simulink model "simu_starting_program23"  (R2023b)
settings: Solver=FixedStepAuto  StartTime=0.0  StopTime=6  RelTol=1e-3
StartFcn:
  | MaxMissedTicks = 99^100;
  | SampleTime = 0.01;
undefined symbols (not defined in the file or in its folder): National_Instruments, PCI
libraries: sldrtlib x24, simulink x2, simulink_extras x2
settings Model: Creator=labadmin  LastModifiedBy=aie4-26
settings HardwareCC: ProdBitPerLong=64  ProdHWDeviceType=Intel->x86-64 (Linux 64)
settings RTWCC: Description=Simulink Desktop Real-Time  SystemTargetFile=sldrt.tlc  TemplateMakefile=sldrt.tmf  RTWCompilerOptimization=on
settings CodeAppCC: MaxIdLength=95
settings SimulinkDesktopRealTimeCC: TargetLibSuffix=_sldrt.a  TargetPreCompLibLocation=C:\Program Files\MATLAB\R2025b\toolbox\sldrt\lib\win64  ParMdlRefBuildCompliant=on
settings ConfigComp: CovBoundaryAbsTol=1.0e-5

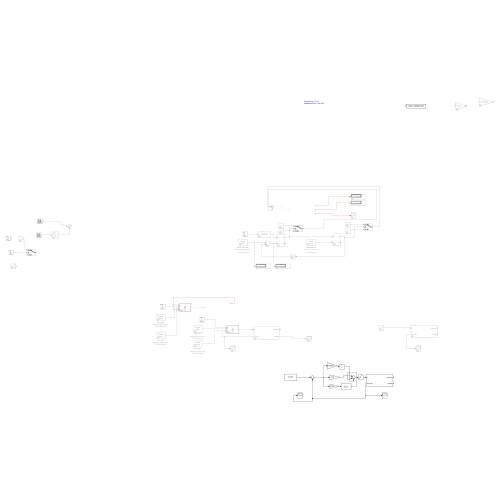
[thumbnail: Simulink's stored preview of the top-level diagram]
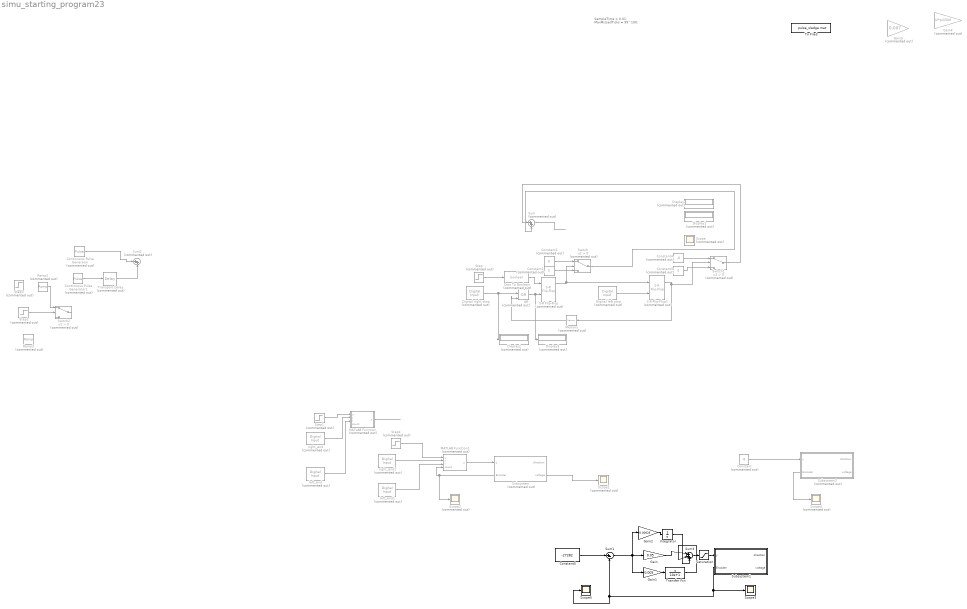
== system simu_starting_program23 ==
  note: SampleTime = 0.01;
      | MaxMissedTicks = 99^100;
  Cast To Boolean : DataTypeConversion  Commented=on  OutDataTypeStr=boolean  SaturateOnIntegerOverflow=off  RndMeth=Floor
  Constant : Constant  Commented=on  Value=-8
  Constant1 : Constant  Commented=on  Value=8
  Constant2 : Constant  Commented=on  Value=0
  Constant3 : Constant  Commented=on  Value=0
  Constant4 : Constant  Commented=on  Value=-8
  Constant5 : Constant  Value=-27282
  Continuous Pulse Generator : DiscretePulseGenerator  Commented=on  PulseType=Time based  Amplitude=1.8  Period=20  PulseWidth=5
  Continuous Pulse Generator1 : DiscretePulseGenerator  Commented=on  PulseType=Time based  Amplitude=-1.8  Period=20  PulseWidth=5
  Digital left stop : sldrtlib/Digital Input  Commented=on  SampleTime=0.1  MaxMissedTicks=10  ShowMissedTicks=off  YieldWhenWaiting=off  DrvName=National_Instruments/PCI-6229  DrvAddress=4294967295  DrvOptions=[1 1 8192 2 3]  Channels=2  BitMode=1  DataType=9
      settings: AttributesFormatString=National Instruments\nPCI-6229 [auto]
  Digital right stop : sldrtlib/Digital Input  Commented=on  SampleTime=0.1  MaxMissedTicks=10  ShowMissedTicks=off  YieldWhenWaiting=off  DrvName=National_Instruments/PCI-6229  DrvAddress=4294967295  DrvOptions=[1 1 8192 2 3]  Channels=3  BitMode=1  DataType=9
      settings: AttributesFormatString=National Instruments\nPCI-6229 [auto]
  Display{,1..3} (4 alike) : Display  Commented=on
  Gain : Gain  Gain=0.05
  Gain1 : Gain  Gain=0.005
  Gain2 : Gain  Gain=0.00026
  Gain4 : Gain  Commented=on  Gain=(2*pi)/500
  Gain5 : Gain  Commented=on  Gain=0.007
  Integrator : Integrator
  MATLAB Function : MATLAB Function  Commented=on  TreatAsAtomicUnit=on
  MATLAB Function1 : MATLAB Function  Commented=on  TreatAsAtomicUnit=on
  Memory : Memory  Commented=on
  OR : Logic  Commented=on  Operator=OR  IconShape=distinctive  AllPortsSameDT=off  OutDataTypeStr=boolean
  Ramp2 : simulink/Sources/Ramp  Commented=on  slope=-2  start=0  InitialOutput=0
  Ramp3 : simulink/Sources/Ramp  Commented=on  slope=1.5  start=7  InitialOutput=0
  S-R Flip-Flop : simulink_extras/Flip Flops/S-R Flip-Flop  Commented=on  initial_condition=0
  S-R Flip-Flop1 : simulink_extras/Flip Flops/S-R Flip-Flop  Commented=on  initial_condition=0
  Saturation : Saturate  UpperLimit=10  LowerLimit=-10
  Scope{,1..2,4} (4 alike) : Scope  Commented=on
  Scope3 : Scope
  Scope5 : Scope
  Step : Step  Commented=on  Before=1  After=0  SampleTime=0
  Step1 : Step  Commented=on  Before=1  After=0  SampleTime=0
  Step2 : Step  Commented=on  Time=6  Before=1  After=0  SampleTime=0
  Step3 : Step  Commented=on  Time=6  Before=1  After=0  SampleTime=0
  Step4 : Step  Commented=on  Before=1  After=0  SampleTime=0
  Subsystem : Subsystem  Commented=on
      settings: PortSchema="{\"entries\":[{\"content\":{\"sides\":[{\"content\":{\"connectorIds\":[\"In1\",\"Out3\"]},\"type\":\"ConnectorPlacement.EquallySpacedRectSide\",\"uuid\":\"4cea31ae-feeb-4317-b838-0a7fffa1c8c1\"},{\"content\":{\"connectorIds\":[\"Out1\",\"Out2\"],\"side\":\"RIGHT\"},\"type\":\"ConnectorPlacement.EquallySpacedRectSide\",\"uuid\":\"cbbf0856-f885-4a01-8596-30b50a35b1ee\"},{\"content\":{\"side\":\"TOP\"},\"type\":\"ConnectorPlacement.EquallySpacedRectSide\",\"uuid\":\"67ac1927-d07b-45dd-8475-804e77d14220\"}]},\"type\":\"ConnectorPlacement.EquallySpacedConnector\",\"uuid\":\"0da884d4-170d-4ce1-a87a-0ec272783a4a\"}],\"packageUris\":[\"http://schema.mathworks.com/mf0/Connector/R2020b\"],\"version\":\"1.0\"}"
  Subsystem1 : Subsystem
      settings: PortSchema="{\"entries\":[{\"content\":{\"sides\":[{\"content\":{\"connectorIds\":[\"In1\",\"Out3\"]},\"type\":\"ConnectorPlacement.EquallySpacedRectSide\",\"uuid\":\"4cea31ae-feeb-4317-b838-0a7fffa1c8c1\"},{\"content\":{\"connectorIds\":[\"Out1\",\"Out2\"],\"side\":\"RIGHT\"},\"type\":\"ConnectorPlacement.EquallySpacedRectSide\",\"uuid\":\"cbbf0856-f885-4a01-8596-30b50a35b1ee\"},{\"content\":{\"side\":\"TOP\"},\"type\":\"ConnectorPlacement.EquallySpacedRectSide\",\"uuid\":\"67ac1927-d07b-45dd-8475-804e77d14220\"}]},\"type\":\"ConnectorPlacement.EquallySpacedConnector\",\"uuid\":\"0da884d4-170d-4ce1-a87a-0ec272783a4a\"}],\"packageUris\":[\"http://schema.mathworks.com/mf0/Connector/R2020b\"],\"version\":\"1.0\"}"
  Subsystem2 : Subsystem  Commented=on
      settings: PortSchema="{\"entries\":[{\"content\":{\"sides\":[{\"content\":{\"connectorIds\":[\"In1\",\"Out3\"]},\"type\":\"ConnectorPlacement.EquallySpacedRectSide\",\"uuid\":\"4cea31ae-feeb-4317-b838-0a7fffa1c8c1\"},{\"content\":{\"connectorIds\":[\"Out1\",\"Out2\"],\"side\":\"RIGHT\"},\"type\":\"ConnectorPlacement.EquallySpacedRectSide\",\"uuid\":\"cbbf0856-f885-4a01-8596-30b50a35b1ee\"},{\"content\":{\"side\":\"TOP\"},\"type\":\"ConnectorPlacement.EquallySpacedRectSide\",\"uuid\":\"67ac1927-d07b-45dd-8475-804e77d14220\"}]},\"type\":\"ConnectorPlacement.EquallySpacedConnector\",\"uuid\":\"0da884d4-170d-4ce1-a87a-0ec272783a4a\"}],\"packageUris\":[\"http://schema.mathworks.com/mf0/Connector/R2020b\"],\"version\":\"1.0\"}"
  Sum : Sum  Commented=on  Inputs=|++
  Sum1 : Sum  Inputs=|+-
  Sum2 : Sum  Commented=on  Inputs=|++
  Sum3 : Sum  Inputs=|+++
  Switch : Switch  Commented=on  Criteria=u2 > Threshold  SaturateOnIntegerOverflow=off  InputSameDT=off
  Switch1 : Switch  Commented=on  Criteria=u2 > Threshold  SaturateOnIntegerOverflow=off  InputSameDT=off
  Switch2 : Switch  Commented=on  Criteria=u2 > Threshold  SaturateOnIntegerOverflow=off  InputSameDT=off
  To File3 : ToFile  Filename=pulse_sledge.mat  SaveFormat=Timeseries
  Transfer Fcn : TransferFcn  Numerator=[1 0 ]  Denominator=[10 1]
  Transport Delay : TransportDelay  Commented=on  DelayTime=10
  left_end : sldrtlib/Digital Input  Commented=on  SampleTime=0.1  MaxMissedTicks=10  ShowMissedTicks=off  YieldWhenWaiting=off  DrvName=National_Instruments/PCI-6229  DrvAddress=4294967295  DrvOptions=[1 1 8192 2 3]  Channels=2  BitMode=1  DataType=1
      settings: AttributesFormatString=National Instruments\nPCI-6229 [auto]
  left_end1 : sldrtlib/Digital Input  Commented=on  SampleTime=0.1  MaxMissedTicks=10  ShowMissedTicks=off  YieldWhenWaiting=off  DrvName=National_Instruments/PCI-6229  DrvAddress=4294967295  DrvOptions=[1 1 8192 2 3]  Channels=2  BitMode=1  DataType=9
      settings: AttributesFormatString=National Instruments\nPCI-6229 [auto]
  right_end : sldrtlib/Digital Input  Commented=on  SampleTime=0.1  MaxMissedTicks=10  ShowMissedTicks=off  YieldWhenWaiting=off  DrvName=National_Instruments/PCI-6229  DrvAddress=4294967295  DrvOptions=[1 1 8192 2 3]  Channels=3  BitMode=1  DataType=9
      settings: AttributesFormatString=National Instruments\nPCI-6229 [auto]
  right_end1 : sldrtlib/Digital Input  Commented=on  SampleTime=0.1  MaxMissedTicks=10  ShowMissedTicks=off  YieldWhenWaiting=off  DrvName=National_Instruments/PCI-6229  DrvAddress=4294967295  DrvOptions=[1 1 8192 2 3]  Channels=3  BitMode=1  DataType=9
      settings: AttributesFormatString=National Instruments\nPCI-6229 [auto]
  wires:
  Continuous Pulse Generator1/1 -> Transport Delay/1
  Continuous Pulse Generator/1 -> Sum2/1
  Transport Delay/1 -> Sum2/2
  Ramp2/1 -> Switch2/1
  Step2/1 -> Switch2/2
  ? -> Display/1
  ? -> Display1/1
  ? -> Scope/1
  Step/1 -> Cast To Boolean/1
  Digital right stop/1 -> Display2/1, OR/1
  OR/1 -> Display3/1, S-R Flip-Flop/2
  S-R Flip-Flop1/1 -> Switch1/2, Memory/1
  S-R Flip-Flop/1 -> S-R Flip-Flop1/1, Switch/2
  Switch/1 -> Sum/2
  Constant2/1 -> Switch/3
  Constant1/1 -> Switch/1
  Constant3/1 -> Switch1/3
  Constant4/1 -> Switch1/1
  Switch1/1 -> Sum/1
  Sum/1 -> ?
  Digital left stop/1 -> S-R Flip-Flop1/2
  Cast To Boolean/1 -> S-R Flip-Flop/1
  Memory/1 -> OR/2
  MATLAB Function/1(y) -> ?
  Step1/1 -> MATLAB Function/1(u)
  right_end/1 -> MATLAB Function/2(r)
  left_end/1 -> MATLAB Function/3(l)
  ? -> MATLAB Function/4(count)
  MATLAB Function1/1(y) -> Subsystem/1(y)
  right_end1/1 -> MATLAB Function1/2(r)
  Step4/1 -> MATLAB Function1/1(u)
  left_end1/1 -> MATLAB Function1/3(l)
  Subsystem/2(voltage) -> Scope1/1
  Subsystem/3(Encoder) -> Scope2/1, MATLAB Function1/4(count)
  Constant5/1 -> Sum1/1
  Gain/1 -> Sum3/1
  Gain1/1 -> Transfer Fcn/1
  Sum3/1 -> Saturation/1
  Constant/1 -> Subsystem2/1(y)
  Subsystem2/3(Encoder) -> Scope4/1
  Sum1/1 -> Gain2/1, Gain1/1, Gain/1
  Subsystem1/3(Encoder) -> Sum1/2, Scope5/1, Scope3/1
  Saturation/1 -> Subsystem1/1(y)
  Transfer Fcn/1 -> Sum3/2
  Gain2/1 -> Integrator/1
  Integrator/1 -> Sum3/3

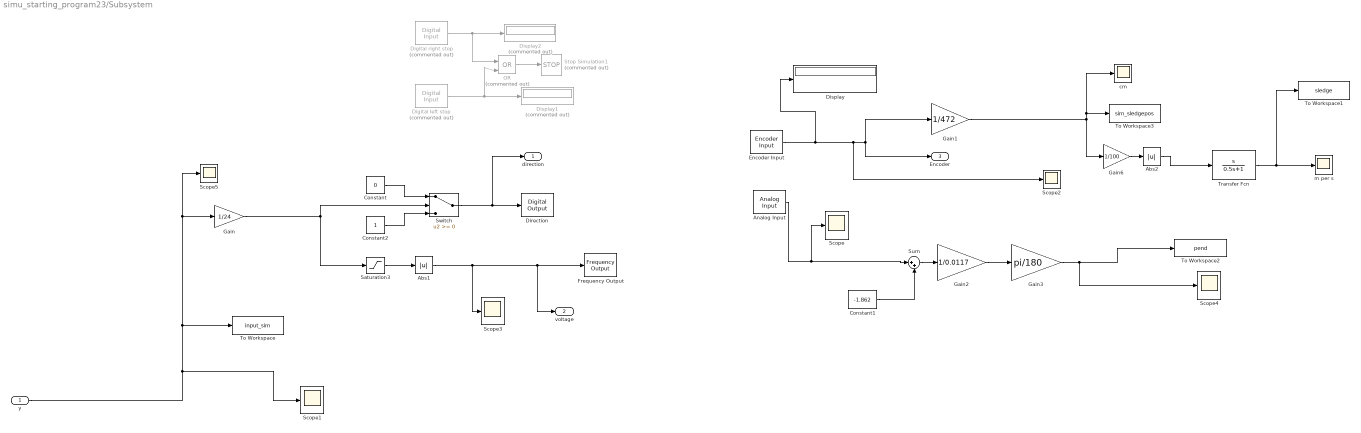
== system simu_starting_program23/Subsystem ==
  y : Inport
  Abs1 : Abs  SaturateOnIntegerOverflow=off
  Abs2 : Abs  SaturateOnIntegerOverflow=off
  Analog Input : sldrtlib/Analog Input  SampleTime=SampleTime  MaxMissedTicks=MaxMissedTicks  ShowMissedTicks=off  YieldWhenWaiting=off  DrvName=National_Instruments/PCI-6229  DrvAddress=4294967295  DrvOptions=[1 1 8192 2 3]  Channels=1  RangeMode=1  VoltRange=1  DataType=1
      settings: AttributesFormatString=National Instruments\nPCI-6229 [auto]
  Constant : Constant  Value=0  SampleTime=SampleTime
  Constant1 : Constant  Value=-1.862
  Constant2 : Constant  SampleTime=SampleTime
  Digital left stop : sldrtlib/Digital Input  Commented=on  SampleTime=0.1  MaxMissedTicks=10  ShowMissedTicks=off  YieldWhenWaiting=off  DrvName=National_Instruments/PCI-6229  DrvAddress=4294967295  DrvOptions=[1 1 8192 2 3]  Channels=2  BitMode=1  DataType=1
      settings: AttributesFormatString=National Instruments\nPCI-6229 [auto]
  Digital right stop : sldrtlib/Digital Input  Commented=on  SampleTime=0.1  MaxMissedTicks=10  ShowMissedTicks=off  YieldWhenWaiting=off  DrvName=National_Instruments/PCI-6229  DrvAddress=4294967295  DrvOptions=[1 1 8192 2 3]  Channels=3  BitMode=1  DataType=9
      settings: AttributesFormatString=National Instruments\nPCI-6229 [auto]
  Direction : sldrtlib/Digital Output  SampleTime=SampleTime  MaxMissedTicks=MaxMissedTicks  ShowMissedTicks=off  YieldWhenWaiting=off  DrvName=National_Instruments/PCI-6229  DrvAddress=4294967295  DrvOptions=[1 1 8192 2 3]  Channels=1  BitMode=1  InitialValue=0  FinalValue=0
      settings: AttributesFormatString=National Instruments\nPCI-6229 [auto]
  Display : Display
  Display1 : Display  Commented=on
  Display2 : Display  Commented=on
  Encoder Input : sldrtlib/Encoder Input  SampleTime=SampleTime  MaxMissedTicks=MaxMissedTicks  ShowMissedTicks=off  YieldWhenWaiting=off  DrvName=National_Instruments/PCI-6229  DrvAddress=4294967295  DrvOptions=[1 1 8192 2 3]  Channels=1  QuadMode=3  IndexPulse=2  InputFilter=Inf  DataType=1
      settings: AttributesFormatString=National Instruments\nPCI-6229 [auto]
  Frequency Output : sldrtlib/Frequency Output  SampleTime=SampleTime  MaxMissedTicks=MaxMissedTicks  ShowMissedTicks=off  YieldWhenWaiting=off  DrvName=National_Instruments/PCI-6229  DrvAddress=4294967295  DrvOptions=[1 1 8192 2 3]  Channels=2  FrequencySource=1  Frequency=10000  FrequencyFinalValue=[]  DutySource=2  Duty=0  DutyFinalValue=0
      settings: AttributesFormatString=National Instruments\nPCI-6229 [auto]
  Gain : Gain  Gain=1/24
  Gain1 : Gain  Gain=1/472
  Gain2 : Gain  Gain=1/0.0117
  Gain3 : Gain  Gain=pi/180
  Gain6 : Gain  Gain=1/100
  OR : Logic  Commented=on  Operator=OR  IconShape=distinctive  AllPortsSameDT=off  OutDataTypeStr=boolean
  Saturation3 : Saturate
  Scope{,1..5} (6 alike) : Scope
  Stop Simulation1 : Stop  Commented=on
  Sum : Sum  Inputs=|++
  Switch : Switch  SaturateOnIntegerOverflow=off  InputSameDT=off
  To Workspace : ToWorkspace  VariableName=input_sim  SaveFormat=Timeseries  SampleTime=-1
  To Workspace1 : ToWorkspace  VariableName=sledge  SaveFormat=Timeseries  SampleTime=-1
  To Workspace2 : ToWorkspace  VariableName=pend  SaveFormat=Timeseries  SampleTime=-1
  To Workspace3 : ToWorkspace  VariableName=sim_sledgepos  SaveFormat=Timeseries  SampleTime=-1
  Transfer Fcn : TransferFcn  Numerator=[1 0]  Denominator=[0.5 1]
  cm : Scope
  m per s : Scope
  direction : Outport
  voltage : Outport  Port=2
  Encoder : Outport  Port=3
  wires:
  Gain1/1 -> Gain6/1, To Workspace3/1, cm/1
  Abs2/1 -> Transfer Fcn/1
  Switch/1 -> direction/1, Direction/1
  Gain2/1 -> Gain3/1
  Digital left stop/1 -> OR/2, Display1/1
  Constant/1 -> Switch/1
  Transfer Fcn/1 -> To Workspace1/1, m per s/1
  y/1 -> To Workspace/1, Scope5/1, Gain/1, Scope1/1
  Gain3/1 -> Scope4/1, To Workspace2/1
  OR/1 -> Stop Simulation1/1
  Digital right stop/1 -> OR/1, Display2/1
  Analog Input/1 -> Sum/1, Scope/1
  Saturation3/1 -> Abs1/1
  Gain/1 -> Saturation3/1, Switch/2
  Gain6/1 -> Abs2/1
  Constant2/1 -> Switch/3
  Sum/1 -> Gain2/1
  Abs1/1 -> Scope3/1, voltage/1, Frequency Output/1
  Constant1/1 -> Sum/2
  Encoder Input/1 -> Display/1, Scope2/1, Encoder/1, Gain1/1

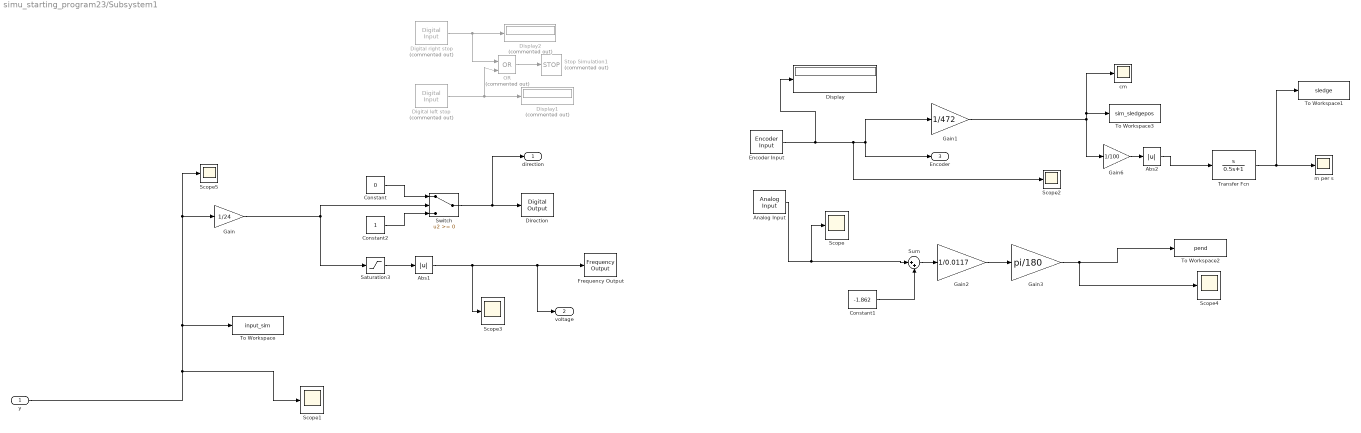
== system simu_starting_program23/Subsystem1 ==
  y : Inport
  Abs1 : Abs  SaturateOnIntegerOverflow=off
  Abs2 : Abs  SaturateOnIntegerOverflow=off
  Analog Input : sldrtlib/Analog Input  SampleTime=SampleTime  MaxMissedTicks=MaxMissedTicks  ShowMissedTicks=off  YieldWhenWaiting=off  DrvName=National_Instruments/PCI-6229  DrvAddress=4294967295  DrvOptions=[1 1 8192 2 3]  Channels=1  RangeMode=1  VoltRange=1  DataType=1
      settings: AttributesFormatString=National Instruments\nPCI-6229 [auto]
  Constant : Constant  Value=0  SampleTime=SampleTime
  Constant1 : Constant  Value=-1.862
  Constant2 : Constant  SampleTime=SampleTime
  Digital left stop : sldrtlib/Digital Input  Commented=on  SampleTime=0.1  MaxMissedTicks=10  ShowMissedTicks=off  YieldWhenWaiting=off  DrvName=National_Instruments/PCI-6229  DrvAddress=4294967295  DrvOptions=[1 1 8192 2 3]  Channels=2  BitMode=1  DataType=1
      settings: AttributesFormatString=National Instruments\nPCI-6229 [auto]
  Digital right stop : sldrtlib/Digital Input  Commented=on  SampleTime=0.1  MaxMissedTicks=10  ShowMissedTicks=off  YieldWhenWaiting=off  DrvName=National_Instruments/PCI-6229  DrvAddress=4294967295  DrvOptions=[1 1 8192 2 3]  Channels=3  BitMode=1  DataType=9
      settings: AttributesFormatString=National Instruments\nPCI-6229 [auto]
  Direction : sldrtlib/Digital Output  SampleTime=SampleTime  MaxMissedTicks=MaxMissedTicks  ShowMissedTicks=off  YieldWhenWaiting=off  DrvName=National_Instruments/PCI-6229  DrvAddress=4294967295  DrvOptions=[1 1 8192 2 3]  Channels=1  BitMode=1  InitialValue=0  FinalValue=0
      settings: AttributesFormatString=National Instruments\nPCI-6229 [auto]
  Display : Display
  Display1 : Display  Commented=on
  Display2 : Display  Commented=on
  Encoder Input : sldrtlib/Encoder Input  SampleTime=SampleTime  MaxMissedTicks=MaxMissedTicks  ShowMissedTicks=off  YieldWhenWaiting=off  DrvName=National_Instruments/PCI-6229  DrvAddress=4294967295  DrvOptions=[1 1 8192 2 3]  Channels=1  QuadMode=3  IndexPulse=2  InputFilter=Inf  DataType=1
      settings: AttributesFormatString=National Instruments\nPCI-6229 [auto]
  Frequency Output : sldrtlib/Frequency Output  SampleTime=SampleTime  MaxMissedTicks=MaxMissedTicks  ShowMissedTicks=off  YieldWhenWaiting=off  DrvName=National_Instruments/PCI-6229  DrvAddress=4294967295  DrvOptions=[1 1 8192 2 3]  Channels=2  FrequencySource=1  Frequency=10000  FrequencyFinalValue=[]  DutySource=2  Duty=0  DutyFinalValue=0
      settings: AttributesFormatString=National Instruments\nPCI-6229 [auto]
  Gain : Gain  Gain=1/24
  Gain1 : Gain  Gain=1/472
  Gain2 : Gain  Gain=1/0.0117
  Gain3 : Gain  Gain=pi/180
  Gain6 : Gain  Gain=1/100
  OR : Logic  Commented=on  Operator=OR  IconShape=distinctive  AllPortsSameDT=off  OutDataTypeStr=boolean
  Saturation3 : Saturate
  Scope{,1..5} (6 alike) : Scope
  Stop Simulation1 : Stop  Commented=on
  Sum : Sum  Inputs=|++
  Switch : Switch  SaturateOnIntegerOverflow=off  InputSameDT=off
  To Workspace : ToWorkspace  VariableName=input_sim  SaveFormat=Timeseries  SampleTime=-1
  To Workspace1 : ToWorkspace  VariableName=sledge  SaveFormat=Timeseries  SampleTime=-1
  To Workspace2 : ToWorkspace  VariableName=pend  SaveFormat=Timeseries  SampleTime=-1
  To Workspace3 : ToWorkspace  VariableName=sim_sledgepos  SaveFormat=Timeseries  SampleTime=-1
  Transfer Fcn : TransferFcn  Numerator=[1 0]  Denominator=[0.5 1]
  cm : Scope
  m per s : Scope
  direction : Outport
  voltage : Outport  Port=2
  Encoder : Outport  Port=3
  wires:
  Encoder Input/1 -> Gain1/1, Encoder/1, Scope2/1, Display/1
  Constant1/1 -> Sum/2
  Abs1/1 -> Frequency Output/1, voltage/1, Scope3/1
  Sum/1 -> Gain2/1
  Constant2/1 -> Switch/3
  Gain6/1 -> Abs2/1
  Gain/1 -> Switch/2, Saturation3/1
  Saturation3/1 -> Abs1/1
  Analog Input/1 -> Scope/1, Sum/1
  Digital right stop/1 -> Display2/1, OR/1
  OR/1 -> Stop Simulation1/1
  Gain3/1 -> To Workspace2/1, Scope4/1
  y/1 -> Scope1/1, Gain/1, Scope5/1, To Workspace/1
  Transfer Fcn/1 -> m per s/1, To Workspace1/1
  Constant/1 -> Switch/1
  Digital left stop/1 -> Display1/1, OR/2
  Gain2/1 -> Gain3/1
  Switch/1 -> Direction/1, direction/1
  Abs2/1 -> Transfer Fcn/1
  Gain1/1 -> cm/1, To Workspace3/1, Gain6/1

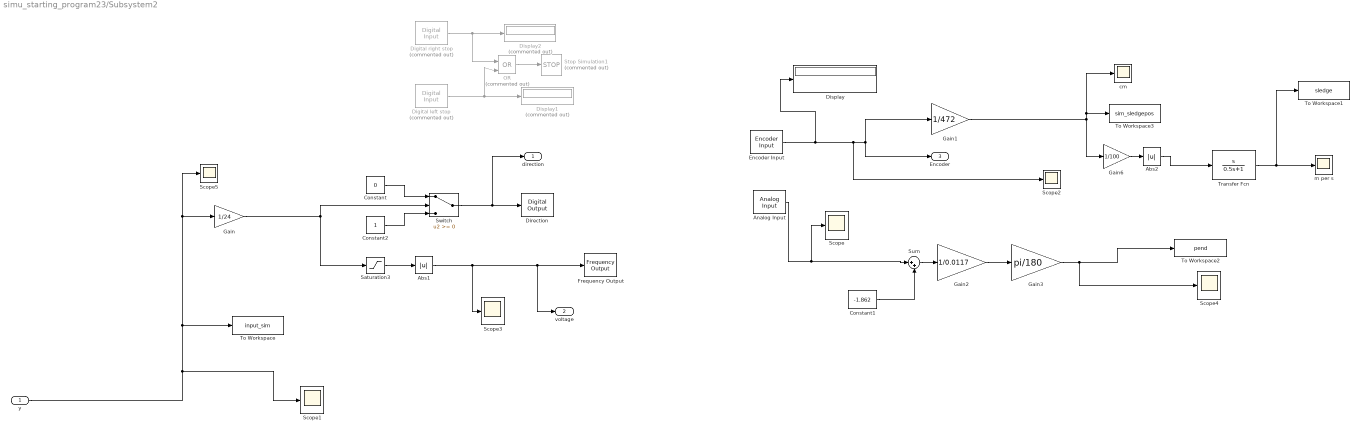
== system simu_starting_program23/Subsystem2 ==
  y : Inport
  Abs1 : Abs  SaturateOnIntegerOverflow=off
  Abs2 : Abs  SaturateOnIntegerOverflow=off
  Analog Input : sldrtlib/Analog Input  SampleTime=SampleTime  MaxMissedTicks=MaxMissedTicks  ShowMissedTicks=off  YieldWhenWaiting=off  DrvName=National_Instruments/PCI-6229  DrvAddress=4294967295  DrvOptions=[1 1 8192 2 3]  Channels=1  RangeMode=1  VoltRange=1  DataType=1
      settings: AttributesFormatString=National Instruments\nPCI-6229 [auto]
  Constant : Constant  Value=0  SampleTime=SampleTime
  Constant1 : Constant  Value=-1.862
  Constant2 : Constant  SampleTime=SampleTime
  Digital left stop : sldrtlib/Digital Input  Commented=on  SampleTime=0.1  MaxMissedTicks=10  ShowMissedTicks=off  YieldWhenWaiting=off  DrvName=National_Instruments/PCI-6229  DrvAddress=4294967295  DrvOptions=[1 1 8192 2 3]  Channels=2  BitMode=1  DataType=1
      settings: AttributesFormatString=National Instruments\nPCI-6229 [auto]
  Digital right stop : sldrtlib/Digital Input  Commented=on  SampleTime=0.1  MaxMissedTicks=10  ShowMissedTicks=off  YieldWhenWaiting=off  DrvName=National_Instruments/PCI-6229  DrvAddress=4294967295  DrvOptions=[1 1 8192 2 3]  Channels=3  BitMode=1  DataType=9
      settings: AttributesFormatString=National Instruments\nPCI-6229 [auto]
  Direction : sldrtlib/Digital Output  SampleTime=SampleTime  MaxMissedTicks=MaxMissedTicks  ShowMissedTicks=off  YieldWhenWaiting=off  DrvName=National_Instruments/PCI-6229  DrvAddress=4294967295  DrvOptions=[1 1 8192 2 3]  Channels=1  BitMode=1  InitialValue=0  FinalValue=0
      settings: AttributesFormatString=National Instruments\nPCI-6229 [auto]
  Display : Display
  Display1 : Display  Commented=on
  Display2 : Display  Commented=on
  Encoder Input : sldrtlib/Encoder Input  SampleTime=SampleTime  MaxMissedTicks=MaxMissedTicks  ShowMissedTicks=off  YieldWhenWaiting=off  DrvName=National_Instruments/PCI-6229  DrvAddress=4294967295  DrvOptions=[1 1 8192 2 3]  Channels=1  QuadMode=3  IndexPulse=2  InputFilter=Inf  DataType=1
      settings: AttributesFormatString=National Instruments\nPCI-6229 [auto]
  Frequency Output : sldrtlib/Frequency Output  SampleTime=SampleTime  MaxMissedTicks=MaxMissedTicks  ShowMissedTicks=off  YieldWhenWaiting=off  DrvName=National_Instruments/PCI-6229  DrvAddress=4294967295  DrvOptions=[1 1 8192 2 3]  Channels=2  FrequencySource=1  Frequency=10000  FrequencyFinalValue=[]  DutySource=2  Duty=0  DutyFinalValue=0
      settings: AttributesFormatString=National Instruments\nPCI-6229 [auto]
  Gain : Gain  Gain=1/24
  Gain1 : Gain  Gain=1/472
  Gain2 : Gain  Gain=1/0.0117
  Gain3 : Gain  Gain=pi/180
  Gain6 : Gain  Gain=1/100
  OR : Logic  Commented=on  Operator=OR  IconShape=distinctive  AllPortsSameDT=off  OutDataTypeStr=boolean
  Saturation3 : Saturate
  Scope{,1..5} (6 alike) : Scope
  Stop Simulation1 : Stop  Commented=on
  Sum : Sum  Inputs=|++
  Switch : Switch  SaturateOnIntegerOverflow=off  InputSameDT=off
  To Workspace : ToWorkspace  VariableName=input_sim  SaveFormat=Timeseries  SampleTime=-1
  To Workspace1 : ToWorkspace  VariableName=sledge  SaveFormat=Timeseries  SampleTime=-1
  To Workspace2 : ToWorkspace  VariableName=pend  SaveFormat=Timeseries  SampleTime=-1
  To Workspace3 : ToWorkspace  VariableName=sim_sledgepos  SaveFormat=Timeseries  SampleTime=-1
  Transfer Fcn : TransferFcn  Numerator=[1 0]  Denominator=[0.5 1]
  cm : Scope
  m per s : Scope
  direction : Outport
  voltage : Outport  Port=2
  Encoder : Outport  Port=3
  wires:
  Gain1/1 -> Gain6/1, To Workspace3/1, cm/1
  Abs2/1 -> Transfer Fcn/1
  Switch/1 -> direction/1, Direction/1
  Gain2/1 -> Gain3/1
  Digital left stop/1 -> OR/2, Display1/1
  Constant/1 -> Switch/1
  Transfer Fcn/1 -> To Workspace1/1, m per s/1
  y/1 -> To Workspace/1, Scope5/1, Gain/1, Scope1/1
  Gain3/1 -> Scope4/1, To Workspace2/1
  OR/1 -> Stop Simulation1/1
  Digital right stop/1 -> OR/1, Display2/1
  Analog Input/1 -> Sum/1, Scope/1
  Saturation3/1 -> Abs1/1
  Gain/1 -> Saturation3/1, Switch/2
  Gain6/1 -> Abs2/1
  Constant2/1 -> Switch/3
  Sum/1 -> Gain2/1
  Abs1/1 -> Scope3/1, voltage/1, Frequency Output/1
  Constant1/1 -> Sum/2
  Encoder Input/1 -> Display/1, Scope2/1, Encoder/1, Gain1/1

== matlab function simu_starting_program23/MATLAB Function1 ==
  settings: updateMethod=DISCRETE
  data: u input; y output; r input; l input; count input
function y = fcn(u, r, l, count)

    persistent step m x subtraction total_count count_length;

    if isempty(step)
        step = 1;
        x = 0;
        m = 0;
        subtraction = false;
        total_count = 0;
        count_length = 0;
    end
   
    
    y = 0;

    if x < 2
        
        if step == 1
            
            y = -8.5;

            if r == 1
                y =0;
                if x == 0
                    m = count;
                end
                pause(0.5)
                x = x+1;
                
                step = 2;
                
            end

        elseif step == 2

            y = 8.5;

            if l == 1
                
                pause(0.5)
                step = 1;
                x = x+1;
                %rounds = rounds + 1;
            end
        
               
           
        end

    else
        y = 0;
        if subtraction == false
            total_count = count - m;
            
            count_length = total_count / 2;
            disp(count_length);
            subtraction = true;
            
        end
    end

end

== matlab function simu_starting_program23/MATLAB Function ==
  data: u input; y output; r input; l input; count input
function y = fcn(u,  r, l, count)
    if u == 0
        while r == false
            y = 8;
